simulink model "VABSim_n_l"  (R2019b)
settings: Solver=FixedStepAuto  StartTime=0.0  StopTime=t_end  FixedStep=Ts  RelTol=1e-3
values from neighbouring files (symbols this model uses):
  alpha = fliplr(poly(A))    [Calcola_T_alpha.m]    (also in fdt_vab_lineare.m = alfa)
  K = [-166015.97989 -40690.286301 -1784658.34431 -399746.424242]    [K.mat]
undefined symbols (not defined in the file or in its folder): control_on, phi_secondo, sigbuilder_block, theta_secondo
settings Model: EnablePacing=on  PacingRate=0.110000  Creator=Michele  LastModifiedBy=AndreaCalegari
settings DataIOCC: ReturnWorkspaceOutputs=off
settings DebuggingCC: StateNameClashWarn=warning  ArithmeticOperatorsInVariantConditions=warning
settings SFSimCC: SimUseLocalCustomCode=off  CustomCodeUndefinedFunction=UseInterfaceOnly
settings RTWCC: RTWUseLocalCustomCode=off
settings CodeAppCC: StateflowObjectComments=on

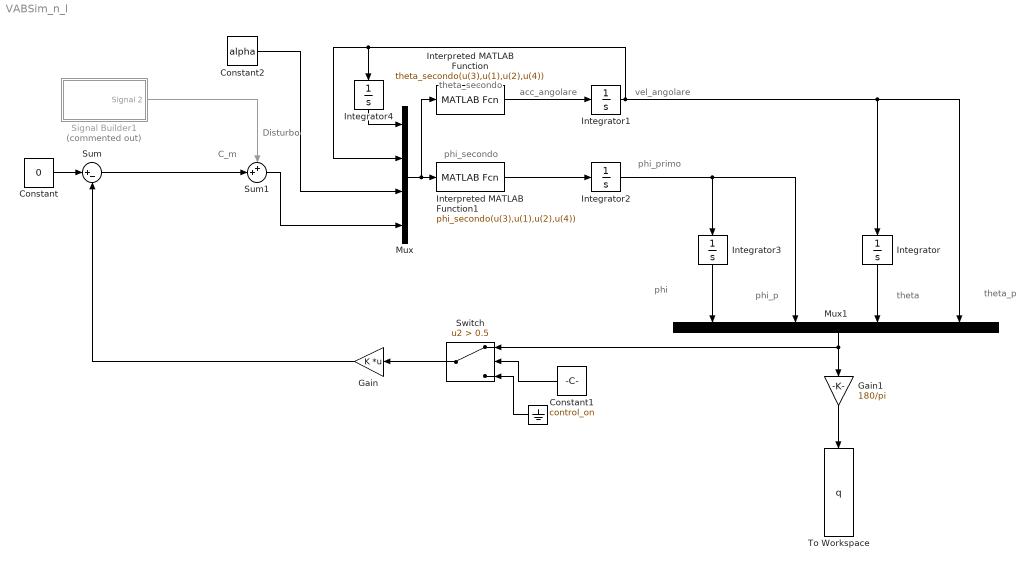
== system VABSim_n_l ==
  note: phi_primo
  note: theta_p
  note: theta
  note: phi_p
  note: phi
  note: phi_secondo
  note: theta_secondo
  note: acc_angolare
  note: vel_angolare
  note: Disturbo
  note: C_m
  " " : Ground
  Constant : Constant  Value=0
  Constant1 : Constant  Value=control_on
  Constant2 : Constant  Value=alpha
  Gain : Gain  Gain=K  Multiplication=Matrix(K*u)
  Gain1 : Gain  Gain=180/pi
  Integrator{,2..4} (4 alike) : Integrator
  Integrator1 : Integrator  UpperSaturationLimit=100  LowerSaturationLimit=-100
  Interpreted MATLAB Function : MATLABFcn  MATLABFcn=theta_secondo(u(3),u(1),u(2),u(4))  OutputDimensions=1
  Interpreted MATLAB Function1 : MATLABFcn  MATLABFcn=phi_secondo(u(3),u(1),u(2),u(4))
  Mux : Mux
  Mux1 : Mux
  Signal Builder1 : Subsystem  Tag=STV Subsys  Commented=on  LoadFcn=sigbuilder_block('load');  StartFcn=sigbuilder_block('start');  StopFcn=sigbuilder_block('stop');  ClipboardFcn=sigbuilder_block('clipboard');  mask(Sigbuilder block){tuvar=[0:10]}
      mask help: Simulink:masks:SigbuilderBlock_MD
      mask init:
      | if ~strcmp(get_param(bdroot(gcbh),'SimulationStatus'),'stopped') tuvar = sigbuilder_block('maskInit'); end
      settings: CopyFcn=sigbuilder_block('copy');  DeleteFcn=sigbuilder_block('delete');  ModelCloseFcn=sigbuilder_block('modelClose');  PreSaveFcn=sigbuilder_block('preSave');  PauseFcn=sigbuilder_block('pause');  ContinueFcn=sigbuilder_block('continue');  NameChangeFcn=sigbuilder_block('namechange');  OpenFcn=sigbuilder_block('open',[6 25.5 1012.5 451.5 ]);  CloseFcn=sigbuilder_block('close');
      mask Display: plot(0, 0, 100, 100,[2, 2, 32, 32, 2], [68, 8, 8, 68, 68],[32, 2], [38, 38], [32, 19, 2],[53, 60, 44], [32, 17, 17, 2],[16, 16, 31, 31]);txt = getActiveGroup(gcbh);text(2, 100, txt,'verticalAlignment', 'top');
  Sum : Sum  Inputs=|+-
  Sum1 : Sum  Inputs=++|
  Switch : Switch  Criteria=u2 > Threshold  Threshold=0.5
  To Workspace : ToWorkspace  VariableName=q  SampleTime=-1
  wires:
  Interpreted MATLAB Function/1 -> Integrator1/1
  Constant/1 -> Sum/1
  Switch/1 -> Gain/1
  Constant1/1 -> Switch/2
  " "/1 -> Switch/3
  Mux/1 -> Interpreted MATLAB Function/1, Interpreted MATLAB Function1/1
  Signal Builder1/1(Signal 2) -> Sum1/1
  Constant2/1 -> Mux/3
  Sum1/1 -> Mux/4
  Sum/1 -> Sum1/2
  Gain/1 -> Sum/2
  Interpreted MATLAB Function1/1 -> Integrator2/1
  Integrator2/1 -> Mux1/2, Integrator3/1
  Integrator3/1 -> Mux1/1
  Integrator1/1 -> Integrator4/1, Mux/2, Mux1/4, Integrator/1
  Integrator/1 -> Mux1/3
  Mux1/1 -> Switch/1, Gain1/1
  Integrator4/1 -> Mux/1
  Gain1/1 -> To Workspace/1

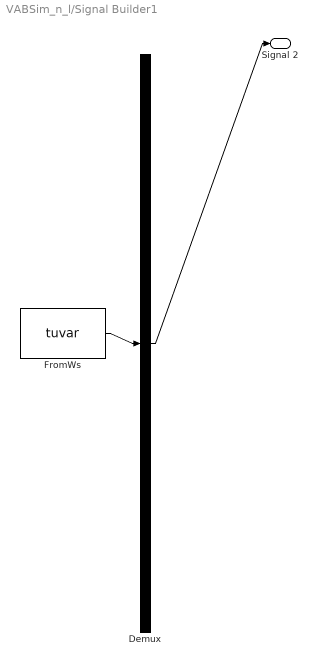
== system VABSim_n_l/Signal Builder1 ==
  Demux : Demux  Tag=STV Demux  Outputs=1
  FromWs : FromWorkspace  Tag=STV FromWs  VariableName=tuvar  SampleTime=0
      SigBuilderData=|
      | common.afterFinalStr = 'Extrapolate'
      | common.sampleTime = 0
      | dataSet.timeRange = [0 20]
      | dataSet.name = 'Group 1'
      | sbobj.Groups.Name = 'Group 1'
      | sbobj.Groups.Signals.Name = 'Signal 2'
      | sbobj.Groups.Signals.XData = [0 8 8 9.96 9.96 20]
      | sbobj.Groups.Signals.YData = [0 0 46.5 46.5 0 0]
      | sbobj.Groups.TimeRange = [0 20]
  Signal 2 : Outport  Tag=STV Outport
  wires:
  FromWs/1 -> Demux/1
  Demux/1 -> Signal 2/1
